simulink model "Mtr_Test02"  (R2022a)
settings: Solver=FixedStepAuto  StartTime=0.0  StopTime=20.0  RelTol=1e-3  EnableMultiTasking=on
libraries: mbedblockslib x6
settings Model: ExtModeTrigDuration=10  Creator=FUGAZI  LastModifiedBy=FUGAZI
settings OptimizationCC: EnhancedBackFolding=on  PassReuseOutputArgsAs=Individual arguments  ZeroExternalMemoryAtStartup=off  ZeroInternalMemoryAtStartup=off  MaxStackSize=64  OptimizeBlockOrder=speed  DifferentSizesBufferReuse=on  OptimizationCustomize=off  EfficientTunableParamExpr=on
settings DebuggingCC: ParameterTunabilityLossMsg=error
settings HardwareCC: ProdBitPerPointer=32  ProdBitPerSizeT=32  ProdBitPerPtrDiffT=32  ProdLargestAtomicInteger=Long  ProdLargestAtomicFloat=Double  ProdWordSize=32  ProdLongLongMode=on  ProdHWDeviceType=ARM Compatible->ARM Cortex
settings SFSimCC: MATLABDynamicMemAlloc=off
settings RTWCC: SystemTargetFile=ert.tlc  HardwareBoard=STM32 Nucleo L476RG  TemplateMakefile=ert_default_tmf  Toolchain=GNU Tools for ARM Embedded Processors
settings CodeAppCC: ForceParamTrailComments=on  IgnoreCustomStorageClasses=off  OperatorAnnotations=on  SimulinkDataObjDesc=on  SFDataObjDesc=on  InsertBlockDesc=on
settings ERTTargetCC: SupportContinuousTime=on  ExtModeTransport=3  ExtModeStaticAlloc=on  ExtModeStaticAllocSize=2000  ExtModeMexFile=ext_xcp  ExtModeIntrfLevel=Level2 - Open

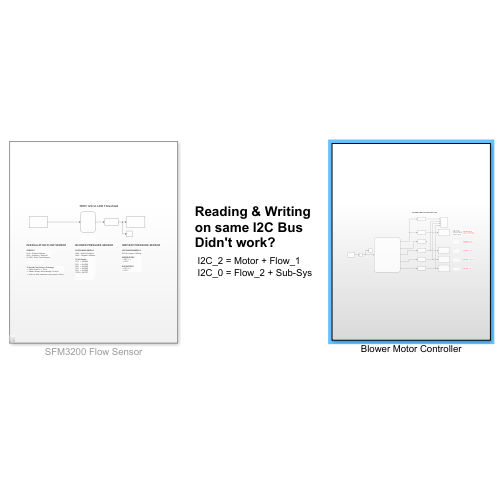
[thumbnail: Simulink's stored preview of the top-level diagram]
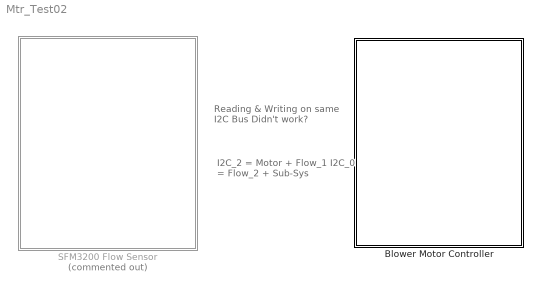
== system Mtr_Test02 ==
  note: Reading & Writing
      | on same I2C Bus
      | Didn't work?
  note: I2C_2 = Motor + Flow_1
      | I2C_0 = Flow_2 + Sub-Sys
  Blower Motor Controller : Subsystem
  SFM3200 Flow Sensor : Subsystem  Commented=on

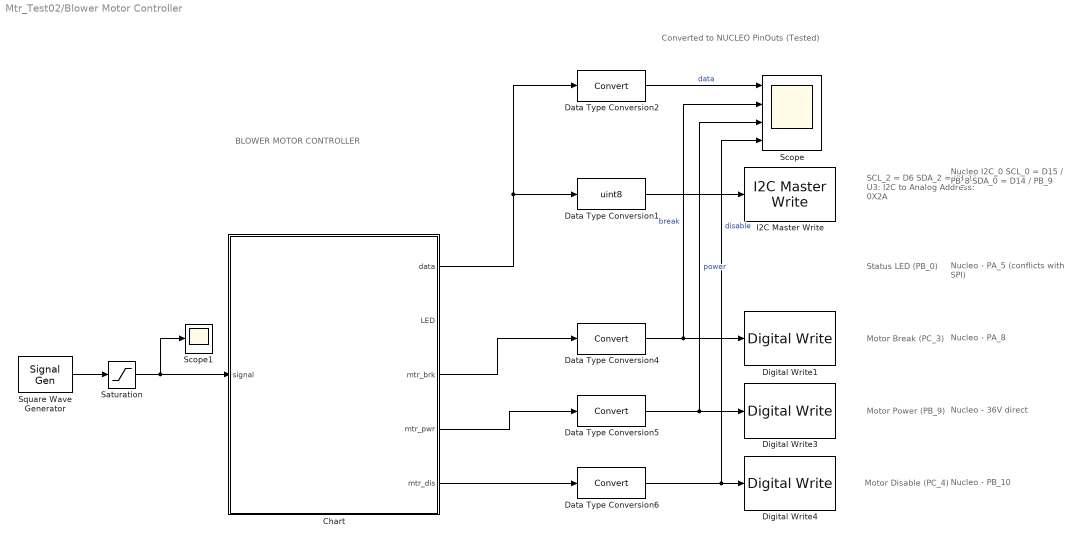
== system Mtr_Test02/Blower Motor Controller ==
  note: Status LED
      | (PB_0)
  note: SCL_2 = D6
      | SDA_2 = PB_11
      | U3: I2C to Analog
      | Address: 0X2A
  note: Converted to NUCLEO PinOuts
      | (Tested)
  note: Motor Break
      | (PC_3)
  note: Motor Power
      | (PB_9)
  note: Motor Disable
      | (PC_4)
  note: Nucleo I2C_0
      | SCL_0 = D15 / PB_8
      | SDA_0 = D14 / PB_9
  note: Nucleo - 36V direct
  note: Nucleo - PA_8
  note: Nucleo - PB_10
  note: Nucleo - PA_5
      | (conflicts with SPI)
  note: BLOWER MOTOR CONTROLLER
  Chart : Stateflow chart  TreatAsAtomicUnit=on
  Data Type Conversion1 : DataTypeConversion  OutDataTypeStr=uint8  SaturateOnIntegerOverflow=off  RndMeth=Floor
  Data Type Conversion{2,4..6} (4 alike) : DataTypeConversion  SaturateOnIntegerOverflow=off  RndMeth=Floor
  Digital Write1 : mbedblockslib/Digital Write  Pin=PA_8  Direction=output
      settings: SourceProductBaseCode=MICROBIT,NUCLEO,STMICRODIS
  Digital Write3 : mbedblockslib/Digital Write  Pin=PB_5  Direction=output
      settings: SourceProductBaseCode=MICROBIT,NUCLEO,STMICRODIS
  Digital Write4 : mbedblockslib/Digital Write  Pin=PB_10  Direction=output
      settings: SourceProductBaseCode=MICROBIT,NUCLEO,STMICRODIS
  I2C Master Write : mbedblockslib/I2C Master Write  I2CModule=0  Mode=Master  SlaveAddress=uint8(hex2dec('2A'))  SlaveByteOrder=BigEndian  Direction=Transmitter  RegisterAddressMode=on  RegisterAddress=uint8(hex2dec('10'))  SlaveDataType=uint8  DataLength=2  NoAck=off  RepeatedStart=off  OutputStatus=off
      settings: SourceProductBaseCode=MICROBIT,NUCLEO,STMICRODIS
  Saturation : Saturate  UpperLimit=250  LowerLimit=0
  Scope : Scope  NumInputPorts=4
  Scope1 : Scope
  Square Wave Generator : SignalGenerator  WaveForm=square  Amplitude=200  Units=rad/sec
  wires:
  Data Type Conversion4/1 -> Scope/2, Digital Write1/1  "break"
  Data Type Conversion5/1 -> Digital Write3/1, Scope/3  "power"
  Chart/1(data) -> Data Type Conversion1/1, Data Type Conversion2/1
  Data Type Conversion2/1 -> Scope/1  "data"
  Chart/3(mtr_brk) -> Data Type Conversion4/1
  Data Type Conversion6/1 -> Scope/4, Digital Write4/1  "disable"
  Chart/4(mtr_pwr) -> Data Type Conversion5/1
  Chart/5(mtr_dis) -> Data Type Conversion6/1
  Data Type Conversion1/1 -> I2C Master Write/1
  Square Wave Generator/1 -> Saturation/1
  Saturation/1 -> Chart/1(signal), Scope1/1

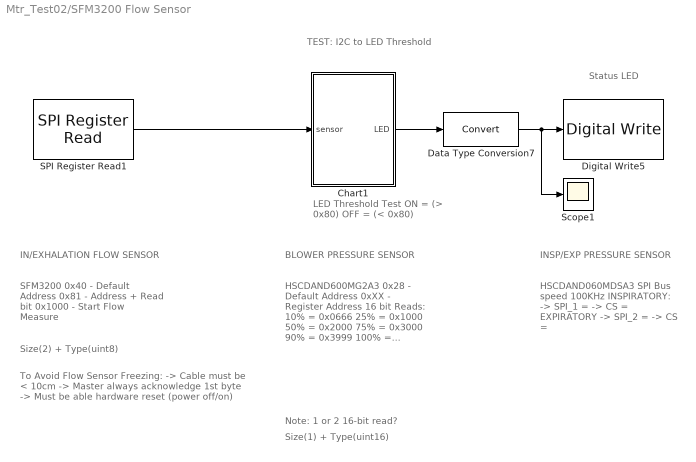
== system Mtr_Test02/SFM3200 Flow Sensor ==
  note: Note: 1 or 2 16-bit read?
  note: LED Threshold Test
      | ON   = (> 0x80)
      | OFF = (< 0x80)
  note: Status LED
  note: IN/EXHALATION FLOW SENSOR
  note: To Avoid Flow Sensor Freezing:
      | -> Cable must be < 10cm
      | -> Master always acknowledge 1st byte
      | -> Must be able hardware reset (power off/on)
  note: TEST: I2C to LED Threshold
  note: SFM3200
      | 0x40 - Default Address
      | 0x81 - Address + Read bit
      | 0x1000 - Start Flow Measure
  note: BLOWER PRESSURE SENSOR
  note: HSCDAND600MG2A3
      | 0x28 - Default Address
      | 0xXX - Register Address
      |
      | 16 bit Reads:
      | 10% = 0x0666
      | 25% = 0x1000
      | 50% = 0x2000
      | 75% = 0x3000
      | 90% = 0x3999
      | 100% = 0x3FFF
  note: Size(2) + Type(uint8)
  note: Size(1) + Type(uint16)
  note: INSP/EXP PRESSURE SENSOR
  note: HSCDAND060MDSA3
      | SPI Bus speed 100KHz
      |
      | INSPIRATORY:
      | -> SPI_1 =
      | -> CS =
      |
      | EXPIRATORY
      | -> SPI_2 =
      | -> CS =
  Chart1 : Stateflow chart  TreatAsAtomicUnit=on
  Data Type Conversion7 : DataTypeConversion  SaturateOnIntegerOverflow=off  RndMeth=Floor
  Digital Write5 : mbedblockslib/Digital Write  Pin=PB_0  Direction=output
      settings: SourceProductBaseCode=MICROBIT,NUCLEO,STMICRODIS
  SPI Register Read1 : mbedblockslib/SPI Register Read  SPIModule=0  Mode=Master  BusSpeed=uint32( 1000000 )  Pin=PA_4  FirstBitToTransfer=Most significant bit (MSB)  ClockMode=0  BlockFunction=Read  RegisterAddress=0  OutputDataType=int16  OutputDataLength=2  SampleTime=0.5  UseCustomSSPin=Explicit GPIO calls  ActiveLowSSPin=Active low
      settings: SourceProductBaseCode=MICROBIT,NUCLEO,STMICRODIS
  Scope1 : Scope
  wires:
  Chart1/1(LED) -> Data Type Conversion7/1
  Data Type Conversion7/1 -> Scope1/1, Digital Write5/1
  SPI Register Read1/1 -> Chart1/1(sensor)

== stateflow chart Mtr_Test02/SFM3200 Flow Sensor/Chart1 ==
  state Check_1
    entry:
    if(sensor >= 0x1000)
    LED = 1;
    else
    LED = 0;
    end
    exit:
  note: Less/Equal to 30%
  note: SPI In/Ex Pressure:
      | 10% = 0x0666
      | 25% = 0x1000
      | 50% = 0x2000
      | 75% = 0x3000
      | 90% = 0x3999
      | 100% = 0x3FFF
  note: I2C Blower Pressure:
      | 10% = 0x0666
      | 25% = 0x1000
      | 50% = 0x2000
      | 75% = 0x3000
      | 90% = 0x3999
      | 100% = 0x3FFF
  state Check_2
    entry:
    if(sensor >= 0x1000)
    LED = 1;
    else
    LED = 0;
    end
    exit:
  (default) -> Check_1
  Check_2 -> Check_1 : after(1,sec)
  Check_1 -> Check_2 : after(1,sec)
  data: LED output; sensor input

== stateflow chart Mtr_Test02/Blower Motor Controller/Chart ==
  state RUN % Startup Sequence
    state Start_1 % Main Power
      entry:
      mtr_dis = 1; % enabled
      LED = 1; % debug
      exit:
    state Start_2 % Motor Brake
      entry:
      mtr_brk = 1; % Disable
      LED = 0; % debug
      exit:
    state Start_3 % Motor Disable
      entry:
      mtr_pwr = 1; % ON
      LED = 1; % debug
      exit:
    state Start_4 % I2C to Anal.
      entry:
      data = signal; % half spd
      LED = 0; % debug
      exit:
    (default) -> Start_1 % Main Power
    Start_1 % Main Power -> Start_2 % Motor Brake : after(1,sec)
    Start_2 % Motor Brake -> Start_3 % Motor Disable : after(1,sec)
    Start_3 % Motor Disable -> Start_4 % I2C to Anal. : after(1,sec)
  state Loop % Continuous Update
    state variable_1 % new data
      entry:
      data = signal;
      LED = 1; % debug
      exit:
    state variable_2 % new data
      entry:
      data = signal;
      LED = 0; % debug
      exit:
    (default) -> variable_1 % new data
    variable_2 % new data -> variable_1 % new data : after(3,sec)
    variable_1 % new data -> variable_2 % new data : after(3,sec)
  state SHUTDOWN % Run-Down
    state Stop_1 % I2C to Anal.
      entry:
      data = 0; % slowest?
      LED = 1;
      exit:
    state Stop_2 % Motor Brake
      entry:
      mtr_dis = 0; % slow
      LED = 0; % debug
      exit:
    state Stop_3 % Motor Disable
      entry:
      mtr_brk = 0; % Enable
      LED = 1; % debug
      exit:
    state Stop_4 % Main Power
      entry:
      mtr_pwr = 0; % OFF
      LED = 0; % debug
      exit:
    (default) -> Stop_1 % I2C to Anal.
    Stop_1 % I2C to Anal. -> Stop_2 % Motor Brake : after(2,sec)
    Stop_2 % Motor Brake -> Stop_3 % Motor Disable : after(1,sec)
    Stop_3 % Motor Disable -> Stop_4 % Main Power : after(2,sec)
  note: Power On first
      | then break & disable?
      | or Power after?
  note: What are all of their
      | initial states?
      | (on power up)
  note: BRAKE PIN:
      | Enabled = <0.8V or Gnd
      | Deactivated = >2.4V or Not wired
  note: DISABLE PIN:
      | Disable = <0.8V or Gnd
      | Enable = >2.4V or Not wired
  note: Speed Values:
      | 0xBF = 3/4 Vout
      | 0x7F = 1/2 Vout
      | 0x40 = 1/4 Vout
  note: LOOP BACK TO START-UP
  (default) -> RUN % Startup Sequence
  RUN % Startup Sequence -> Loop % Continuous Update : after(5, sec)
  Loop % Continuous Update -> SHUTDOWN % Run-Down : after(35,sec)
  data: data output; LED output; mtr_brk output; mtr_pwr output; mtr_dis output; signal input
